simulink model "w14_vitri_vantoc_giatoc"  (R2018a)
settings: Solver=VariableStepAuto  StartTime=0.0  StopTime=15  RelTol=1e-3
values from neighbouring files (symbols this model uses):
  Im = 0.01    [Parameters.m]    (also in Parameters.mat = 2; parametersAcc.m; parametersPos.m; parametersVel.m)
  KA = 2    [Parameters.m]    (also in Parameters.mat; parametersAcc.m = 1.5)
  KP = 5    [Parameters.m]    (also in Parameters.mat; parametersAcc.m = 26; parametersPos.m; parametersVel.m)
  kt = 2    [Parameters.m]    (also in Parameters.mat; parametersAcc.m; parametersPos.m; parametersVel.m)
  kTA = 1    [Parameters.m]    (also in Parameters.mat; parametersAcc.m)
  kTP = 1    [Parameters.m]    (also in Parameters.mat; parametersAcc.m; parametersPos.m; parametersVel.m)
  kTV = 1    [Parameters.m]    (also in Parameters.mat; parametersAcc.m; parametersVel.m)
  KV = 10    [Parameters.m]    (also in Parameters.mat; parametersAcc.m = 12; parametersVel.m)
  kv = 2    [Parameters.m]    (also in Parameters.mat; parametersAcc.m; parametersPos.m; parametersVel.m)
  Ra = 10    [Parameters.m]    (also in Parameters.mat; parametersAcc.m; parametersPos.m; parametersVel.m)
  TA = 0    [Parameters.m]    (also in Parameters.mat = 5; parametersAcc.m = 0.025)
libraries: simulink x1
settings Model: Creator=Nguyen Mai  LastModifiedBy=Nguyen Mai

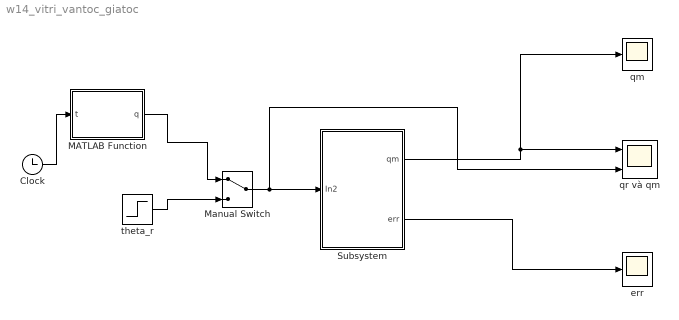
== system w14_vitri_vantoc_giatoc ==
  Clock : Clock
      settings: Decimation=100
  MATLAB Function : MATLAB Function  TreatAsAtomicUnit=on
  Manual Switch : ManualSwitch
  Subsystem : Subsystem
  "err " : Scope
  "qm " : Scope
  qr và qm : Scope  NumInputPorts=2
  theta_r : Step  SampleTime=0
  wires:
  theta_r/1 -> Manual Switch/2
  MATLAB Function/1(q) -> Manual Switch/1
  Clock/1 -> MATLAB Function/1(t)
  Manual Switch/1 -> qr và qm/2, Subsystem/1(In2)
  Subsystem/1(qm) -> "qm "/1, qr và qm/1
  Subsystem/2(err) -> "err "/1

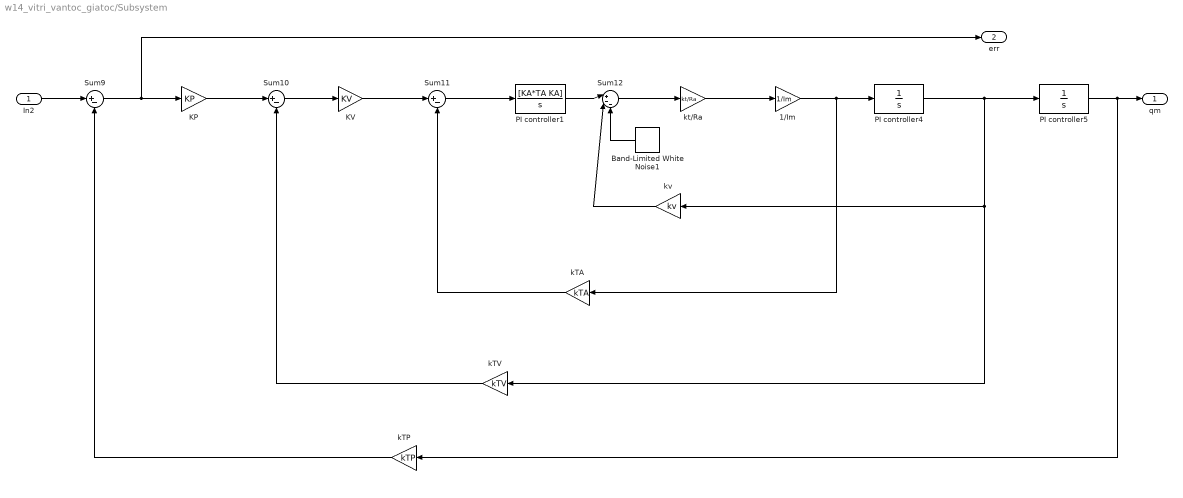
== system w14_vitri_vantoc_giatoc/Subsystem ==
  In2 : Inport
  1/Im : Gain  Gain=1/Im
  Band-Limited White Noise1 : simulink/Sources/Band-Limited White Noise  Cov=[0.1]  Ts=0.1  seed=[23341]
  KP : Gain  Gain=KP
  KV : Gain  Gain=KV
  PI controller1 : TransferFcn  Numerator=[KA*TA KA]  Denominator=[1 0]
  PI controller4 : TransferFcn  Numerator=[0 1]  Denominator=[1 0]
  PI controller5 : TransferFcn  Numerator=[0 1]  Denominator=[1 0]
  Sum10 : Sum  Inputs=|+-
  Sum11 : Sum  Inputs=|+-
  Sum12 : Sum  Inputs=|+--
  Sum9 : Sum  Inputs=|+-
  kTA : Gain  Gain=kTA
  kTP : Gain  Gain=kTP
  kTV : Gain  Gain=kTV
  kt/Ra : Gain  Gain=kt/Ra
  kv : Gain  Gain=kv
  qm : Outport
  err : Outport  Port=2
  wires:
  KV/1 -> Sum11/1
  In2/1 -> Sum9/1
  Sum9/1 -> err/1, KP/1
  KP/1 -> Sum10/1
  Sum10/1 -> KV/1
  Sum11/1 -> PI controller1/1
  PI controller1/1 -> Sum12/1
  Sum12/1 -> kt/Ra/1
  kt/Ra/1 -> 1/Im/1
  1/Im/1 -> kTA/1, PI controller4/1
  PI controller4/1 -> kv/1, kTV/1, PI controller5/1
  PI controller5/1 -> kTP/1, qm/1
  kTP/1 -> Sum9/2
  kTV/1 -> Sum10/2
  kTA/1 -> Sum11/2
  kv/1 -> Sum12/2
  Band-Limited White Noise1/1 -> Sum12/3

== matlab function w14_vitri_vantoc_giatoc/MATLAB Function ==
  data: t input; q output
function q = fcn(t)
t0=0;
tf=40;
tc=4/5;
if t<tc
q=40+(125/8)*t^2;
else
if t<tf-tc
q=30+25*t;
else
q=1020-(125/8)*(40-t)^2;
end
end
